simulink model "WaterFlowSubsystem"  (R2024b)
settings: Solver=ode1  StartTime=0.0  StopTime=5  RelTol=1e-3
values from neighbouring files (symbols this model uses):
  N_l_limit = 15    [rinsing.m]    (also in soaking.m; washing.m = 25)
  N_u_limit = 25    [rinsing.m]    (also in soaking.m; washing.m = 75)
  Water_switch = 1    [rinsing.m]    (also in soaking.m; washing.m)
libraries: simulink x2
settings Model: PacingRate=0.280000  Creator=edine  LastModifiedBy=edine

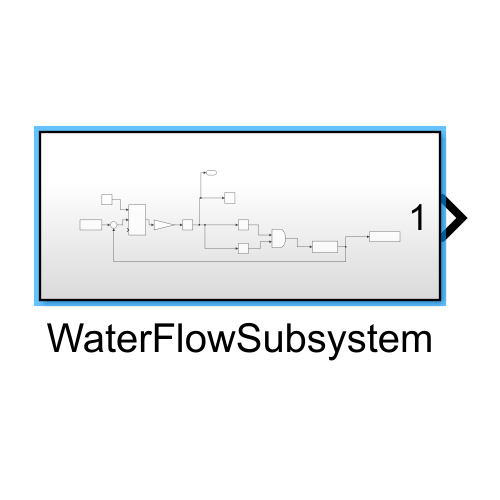
[thumbnail: Simulink's stored preview of the top-level diagram]
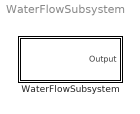
== system WaterFlowSubsystem ==
  WaterFlowSubsystem : Subsystem

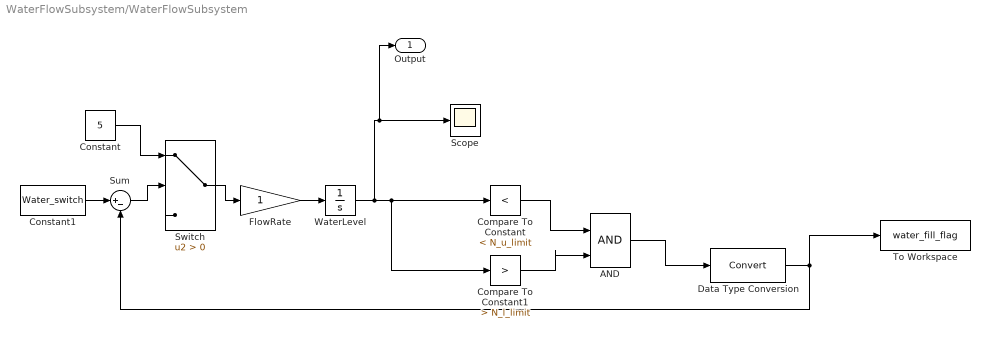
== system WaterFlowSubsystem/WaterFlowSubsystem ==
  AND : Logic  IconShape=distinctive  AllPortsSameDT=off  OutDataTypeStr=boolean
  Compare To Constant : simulink/Logic and Bit Operations/Compare To Constant  relop=<  const=N_u_limit  OutDataTypeStr=boolean
  Compare To Constant1 : simulink/Logic and Bit Operations/Compare To Constant  relop=>  const=N_l_limit  OutDataTypeStr=boolean
  Constant : Constant  Value=5
  Constant1 : Constant  Value=Water_switch
  Data Type Conversion : DataTypeConversion  SaturateOnIntegerOverflow=off  RndMeth=Floor
  FlowRate : Gain
  Scope : Scope
  Sum : Sum  Inputs=|+-
  Switch : Switch  Criteria=u2 > Threshold  SaturateOnIntegerOverflow=off  InputSameDT=off
  To Workspace : ToWorkspace  VariableName=water_fill_flag  SaveFormat=Structure  SampleTime=-1
      settings: Save2DSignal=2-D array (concatenate along first dimension)
  WaterLevel : Integrator
  Output : Outport
  wires:
  FlowRate/1 -> WaterLevel/1
  WaterLevel/1 -> Compare To Constant/1, Compare To Constant1/1, Output/1, Scope/1
  Constant/1 -> Switch/1
  Switch/1 -> FlowRate/1
  Sum/1 -> Switch/2
  Constant1/1 -> Sum/1
  Compare To Constant/1 -> AND/1
  Compare To Constant1/1 -> AND/2
  AND/1 -> Data Type Conversion/1
  Data Type Conversion/1 -> Sum/2, To Workspace/1
